simulink model "Task3Lab7Cs"  (R2015a)
settings: Solver=ode45  StartTime=0.0  StopTime=100.0  RelTol=1e-3
settings Model: Creator=Quswar Mahmood Abid  LastModifiedBy=Quswar Mahmood Abid

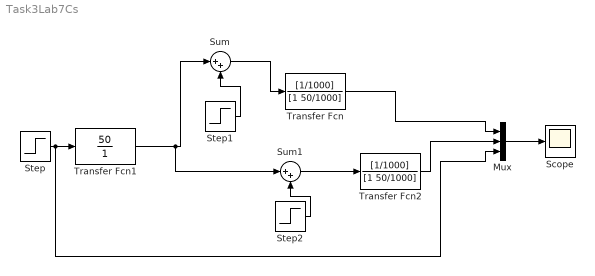
== system Task3Lab7Cs ==
  Mux : Mux  Inputs=3
  Scope : Scope
  Step : Step  Time=0  After=500  SampleTime=0
  Step1 : Step  Time=0  After=2000  SampleTime=0
  Step2 : Step  Time=0  After=6000  SampleTime=0
  Sum : Sum  Inputs=|++
  Sum1 : Sum  Inputs=|++
  Transfer Fcn : TransferFcn  Numerator=[1/1000]  Denominator=[1 50/1000]
  Transfer Fcn1 : TransferFcn  Numerator=[50]  Denominator=[1]
  Transfer Fcn2 : TransferFcn  Numerator=[1/1000]  Denominator=[1 50/1000]
  wires:
  Step/1 -> Transfer Fcn1/1, Mux/3
  Transfer Fcn1/1 -> Sum/1, Sum1/1
  Sum/1 -> Transfer Fcn/1
  Step1/1 -> Sum/2
  Step2/1 -> Sum1/2
  Sum1/1 -> Transfer Fcn2/1
  Transfer Fcn/1 -> Mux/1
  Transfer Fcn2/1 -> Mux/2
  Mux/1 -> Scope/1
